simulink model "ArduinoDUE"  (R2024b)
settings: Solver=ode3  StartTime=0.0  StopTime=inf  RelTol=1e-3  EnableMultiTasking=on
libraries: arduinolib x7, simulink x5, arduinosensorlib x2, slpidlib x2
settings Model: SimulationMode=external  ExtModeTrigDuration=2  Creator=antho  LastModifiedBy=antho
settings SolverCC: AlgebraicLoopSolver=TrustRegion  AutoInsertRateTranBlk=on
settings DataIOCC: LimitDataPoints=on  SaveFormat=Array
settings OptimizationCC: ReuseModelBlockBuffer=off  ExpressionDepthLimit=2147483647  LifeSpan=Inf  MaxStackSize=64
settings DebuggingCC: UnderspecifiedInitializationDetection=Classic  MergeDetectMultiDrivingBlocksExec=none  FcnCallInpInsideContextMsg=warning  UnconnectedInputMsg=warning  UnconnectedOutputMsg=warning  UnconnectedLineMsg=warning  AllowSymbolicDim=off  StateNameClashWarn=warning  SFUnexpectedBacktrackingDiag=warning  SFNoUnconditionalDefaultTransitionDiag=warning  SFExecutionAtInitializationDiag=none  ArithmeticOperatorsInVariantConditions=warning
settings HardwareCC: ProdBitPerPointer=32  ProdBitPerSizeT=32  ProdBitPerPtrDiffT=32  ProdLargestAtomicInteger=Long  ProdLargestAtomicFloat=Double  ProdWordSize=32  ProdHWDeviceType=ARM Compatible->ARM Cortex
settings ModelReferenceCC: EnableRefExpFcnMdlSchedulingChecks=on  PropagateSignalLabelsOutOfModel=off
settings SFSimCC: SimUseLocalCustomCode=off  CustomCodeUndefinedFunction=UseInterfaceOnly
settings RTWCC: Description=Embedded Coder  SystemTargetFile=ert.tlc  HardwareBoard=Arduino Due  TemplateMakefile=ert_default_tmf  GenerateReport=on  RTWVerbose=off  RTWUseLocalCustomCode=off  Toolchain=Arduino ARM  BuildConfiguration=Faster Runs  LaunchReport=on  GPUComputeCapability=3.5
settings CodeAppCC: ForceParamTrailComments=on  OperatorAnnotations=on  StateflowObjectComments=on  MATLABSourceComments=on
settings ERTTargetCC: MultiwordLength=2048  ERTCustomFileBanners=off  SupportContinuousTime=on  SupportNonInlinedSFcns=on  RemoveResetFunc=off  SupportVariableSizeSignals=on  ModelStepFunctionPrototypeControlCompliant=off  ExtModeTransport=3  ExtModeStaticAlloc=on  ExtModeAutomaticAllocSize=off  ExtModeStaticAllocSize=24576  ExtModeMexFile=ext_xcp  ExtModeIntrfLevel=Level2 - Open  InlinedParameterPlacement=Hierarchical  DynamicArrayContainerType=coder::array
settings ConfigComp: CovMetricSettings=dw  CovSaveCumulativeToWorkspaceVar=on  CovSaveSingleToWorkspaceVar=on  CovExternalEMLEnable=off  CovSFcnEnable=off

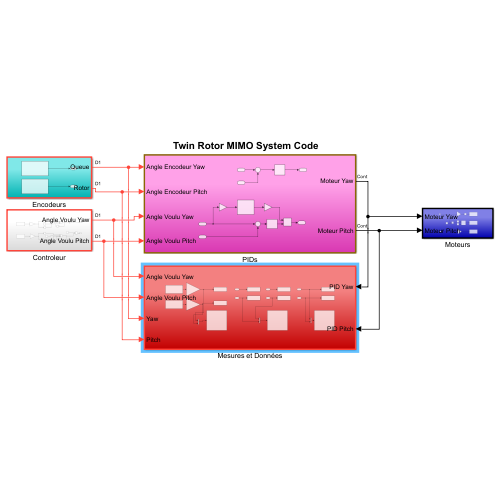
[thumbnail: Simulink's stored preview of the top-level diagram]
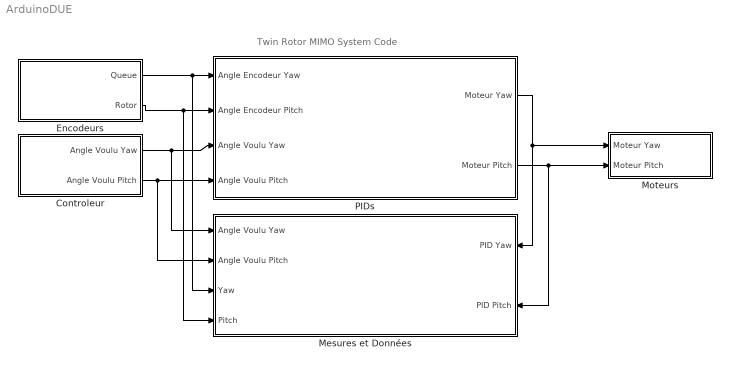
== system ArduinoDUE ==
  note: Twin Rotor MIMO System Code
  Controleur : Subsystem
  Encodeurs : Subsystem
  Mesures et Données : Subsystem
      settings: PortSchema="{\"entries\":[{\"content\":{\"sides\":[{\"content\":{\"connectorIds\":[\"In1\",\"In2\",\"In3\",\"In4\"]},\"type\":\"ConnectorPlacement.EquallySpacedRectSide\",\"uuid\":\"82e4522a-b4cd-44f9-a5c9-60d23544d279\"},{\"content\":{\"connectorIds\":[\"In5\",\"In6\"],\"side\":\"RIGHT\"},\"type\":\"ConnectorPlacement.EquallySpacedRectSide\",\"uuid\":\"29cf5c3e-0c08-4941-86a4-f83772340204\"},{\"content\":{\"side\":\"TOP\"},\"type\":\"ConnectorPlacement.EquallySpacedRectSide\",\"uuid\":\"e18b2821-c2fe-4315-852d-b03618fbc173\"}]},\"type\":\"ConnectorPlacement.EquallySpacedConnector\",\"uuid\":\"8888ef34-2317-47d3-9079-024b33e04ca1\"}],\"packageUris\":[\"http://schema.mathworks.com/mf0/Connector/R2020b\"],\"version\":\"1.0\"}"
  Moteurs : Subsystem
  PIDs : Subsystem
  wires:
  Encodeurs/1(Queue) -> Mesures et Données/3(Yaw), PIDs/1(Angle Encodeur Yaw)
  Encodeurs/2(Rotor) -> Mesures et Données/4(Pitch), PIDs/2(Angle Encodeur Pitch)
  Controleur/1(Angle Voulu Yaw) -> Mesures et Données/1(Angle Voulu Yaw), PIDs/3(Angle Voulu Yaw)
  Controleur/2(Angle Voulu Pitch) -> Mesures et Données/2(Angle Voulu Pitch), PIDs/4(Angle Voulu Pitch)
  PIDs/1(Moteur Yaw) -> Moteurs/1(Moteur Yaw), Mesures et Données/5(PID Yaw)
  PIDs/2(Moteur Pitch) -> Mesures et Données/6(PID Pitch), Moteurs/2(Moteur Pitch)

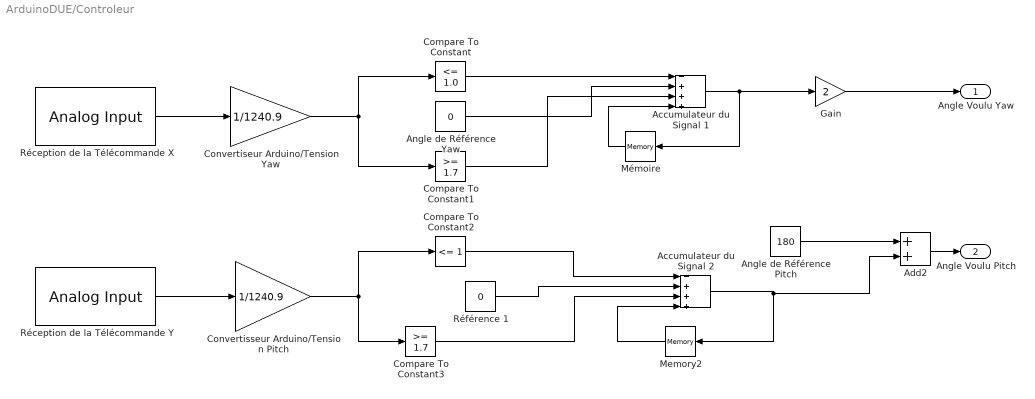
== system ArduinoDUE/Controleur ==
  Accumulateur du Signal 1 : Sum  Inputs=-+++
  Accumulateur du Signal 2 : Sum  Inputs=-+++
  Add2 : Sum
  Angle de Référence Pitch : Constant  Value=180
  Angle de Référence Yaw : Constant  Value=0
  Compare To Constant : simulink/Logic and Bit Operations/Compare To Constant  relop=<=  const=1.0  OutDataTypeStr=boolean
  Compare To Constant1 : simulink/Logic and Bit Operations/Compare To Constant  relop=>=  const=1.7  OutDataTypeStr=boolean
  Compare To Constant2 : simulink/Logic and Bit Operations/Compare To Constant  relop=<=  const=1  OutDataTypeStr=boolean
  Compare To Constant3 : simulink/Logic and Bit Operations/Compare To Constant  relop=>=  const=1.7  OutDataTypeStr=boolean
  Convertiseur Arduino/Tension Yaw : Gain  Gain=1/1240.9
  Convertisseur Arduino/Tension Pitch : Gain  Gain=1/1240.9
  Gain : Gain  Gain=2
  Memory2 : Memory
  Mémoire : Memory
  Réception de la Télécommande X : arduinolib/Analog Input  pinNumber=3  ReadResultsOnly=off  ConversionTriggerSource=Software  ExternalTriggerType=uint32( 0 )  OutputDataType=uint16  EnableConversionCompleteNotify=off  EnableOuputStatus=off  SampleTime=0.005  blockPlatform=arduino
  Réception de la Télécommande Y : arduinolib/Analog Input  pinNumber=4  ReadResultsOnly=off  ConversionTriggerSource=Software  ExternalTriggerType=uint32( 0 )  OutputDataType=uint16  EnableConversionCompleteNotify=off  EnableOuputStatus=off  SampleTime=0.005  blockPlatform=arduino
  Référence 1 : Constant  Value=0
  Angle Voulu Yaw : Outport
  Angle Voulu Pitch : Outport  Port=2
  wires:
  Convertiseur Arduino/Tension Yaw/1 -> Compare To Constant/1, Compare To Constant1/1
  Réception de la Télécommande Y/1 -> Convertisseur Arduino/Tension Pitch/1
  Convertisseur Arduino/Tension Pitch/1 -> Compare To Constant2/1, Compare To Constant3/1
  Réception de la Télécommande X/1 -> Convertiseur Arduino/Tension Yaw/1
  Accumulateur du Signal 1/1 -> Gain/1, Mémoire/1
  Angle de Référence Pitch/1 -> Add2/1
  Mémoire/1 -> Accumulateur du Signal 1/4
  Angle de Référence Yaw/1 -> Accumulateur du Signal 1/2
  Référence 1/1 -> Accumulateur du Signal 2/2
  Memory2/1 -> Accumulateur du Signal 2/4
  Accumulateur du Signal 2/1 -> Add2/2, Memory2/1
  Add2/1 -> Angle Voulu Pitch/1
  Compare To Constant/1 -> Accumulateur du Signal 1/1
  Compare To Constant2/1 -> Accumulateur du Signal 2/1
  Compare To Constant3/1 -> Accumulateur du Signal 2/3
  Compare To Constant1/1 -> Accumulateur du Signal 1/3
  Gain/1 -> Angle Voulu Yaw/1

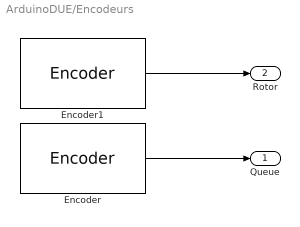
== system ArduinoDUE/Encodeurs ==
  Encoder : arduinosensorlib/Encoder  InputA=3  InputB=2  Mode=No reset  SampleTime=0.005
  Encoder1 : arduinosensorlib/Encoder  InputA=4  InputB=5  Mode=No reset  SampleTime=0.005
  Queue : Outport
  Rotor : Outport  Port=2
  wires:
  Encoder/1 -> Queue/1
  Encoder1/1 -> Rotor/1

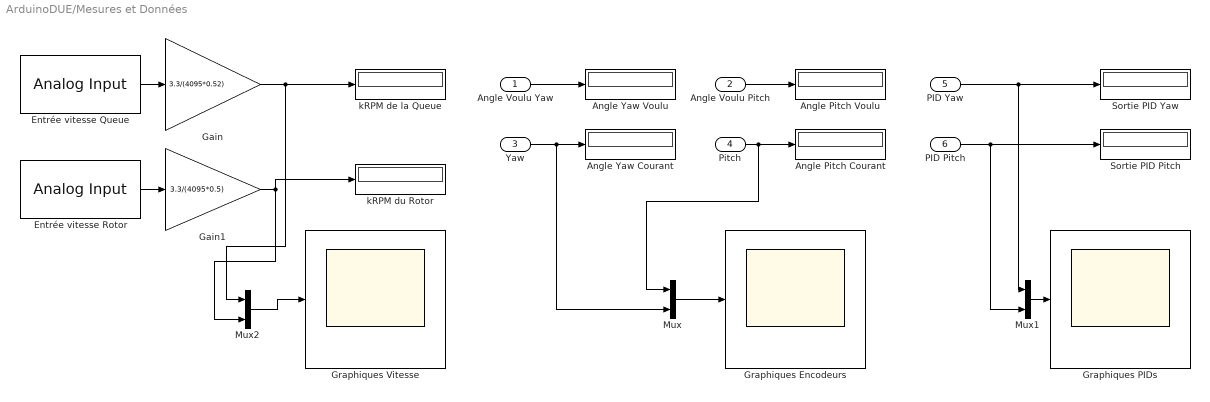
== system ArduinoDUE/Mesures et Données ==
  Angle Voulu Yaw : Inport
  Angle Voulu Pitch : Inport  Port=2
  Yaw : Inport  Port=3
  Pitch : Inport  Port=4
  PID Yaw : Inport  Port=5
  PID Pitch : Inport  Port=6
  Angle Pitch Courant : Display
  Angle Pitch Voulu : Display
  Angle Yaw Courant : Display
  Angle Yaw Voulu : Display
  Entrée vitesse Queue : arduinolib/Analog Input  pinNumber=2  ReadResultsOnly=off  ConversionTriggerSource=Software  ExternalTriggerType=uint32( 0 )  OutputDataType=uint16  EnableConversionCompleteNotify=off  EnableOuputStatus=off  SampleTime=0.005  blockPlatform=arduino
  Entrée vitesse Rotor : arduinolib/Analog Input  pinNumber=1  ReadResultsOnly=off  ConversionTriggerSource=Software  ExternalTriggerType=uint32( 0 )  OutputDataType=uint16  EnableConversionCompleteNotify=off  EnableOuputStatus=off  SampleTime=0.005  blockPlatform=arduino
  Gain : Gain  Gain=3.3/(4095*0.52)
  Gain1 : Gain  Gain=3.3/(4095*0.5)
  Graphiques Encodeurs : Scope
  Graphiques PIDs : Scope
  Graphiques Vitesse : Scope
  Mux : Mux  Inputs=2
  Mux1 : Mux  Inputs=2
  Mux2 : Mux  Inputs=2
  Sortie PID Pitch : Display
  Sortie PID Yaw : Display
  kRPM de la Queue : Display
  kRPM du Rotor : Display
  wires:
  Angle Voulu Yaw/1 -> Angle Yaw Voulu/1
  Yaw/1 -> Mux/2, Angle Yaw Courant/1
  Angle Voulu Pitch/1 -> Angle Pitch Voulu/1
  Pitch/1 -> Mux/1, Angle Pitch Courant/1
  PID Yaw/1 -> Mux1/1, Sortie PID Yaw/1
  PID Pitch/1 -> Mux1/2, Sortie PID Pitch/1
  Mux/1 -> Graphiques Encodeurs/1
  Entrée vitesse Queue/1 -> Gain/1
  Entrée vitesse Rotor/1 -> Gain1/1
  Mux1/1 -> Graphiques PIDs/1
  Mux2/1 -> Graphiques Vitesse/1
  Gain/1 -> Mux2/1, kRPM de la Queue/1
  Gain1/1 -> Mux2/2, kRPM du Rotor/1

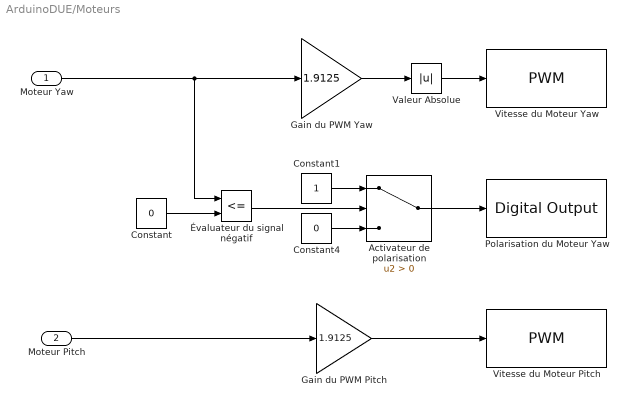
== system ArduinoDUE/Moteurs ==
  Moteur Yaw : Inport
  Moteur Pitch : Inport  Port=2
  Activateur de polarisation : Switch  Criteria=u2 > Threshold  SaturateOnIntegerOverflow=off  InputSameDT=off
  Constant : Constant  Value=0
  Constant1 : Constant
  Constant4 : Constant  Value=0
  Gain du PWM Pitch : Gain  Gain=1.9125
  Gain du PWM Yaw : Gain  Gain=1.9125
  Polarisation du Moteur Yaw : arduinolib/Digital Output  pinNumber=8  Direction=output  blockPlatform=arduino
  Valeur Absolue : Abs  SaturateOnIntegerOverflow=off
  Vitesse du Moteur Pitch : arduinolib/PWM  pinNumber=7  frequencyType=Specify  desiredFrequency=60  achievableFrequency=60
  Vitesse du Moteur Yaw : arduinolib/PWM  pinNumber=6  frequencyType=Specify  desiredFrequency=60  achievableFrequency=60
  Évaluateur du signal négatif : RelationalOperator  Operator=<=  OutDataTypeStr=boolean  RndMeth=Simplest  InputSameDT=off
  wires:
  Évaluateur du signal négatif/1 -> Activateur de polarisation/2
  Constant4/1 -> Activateur de polarisation/3
  Constant1/1 -> Activateur de polarisation/1
  Activateur de polarisation/1 -> Polarisation du Moteur Yaw/1
  Constant/1 -> Évaluateur du signal négatif/2
  Gain du PWM Yaw/1 -> Valeur Absolue/1
  Valeur Absolue/1 -> Vitesse du Moteur Yaw/1
  Moteur Yaw/1 -> Évaluateur du signal négatif/1, Gain du PWM Yaw/1
  Moteur Pitch/1 -> Gain du PWM Pitch/1
  Gain du PWM Pitch/1 -> Vitesse du Moteur Pitch/1

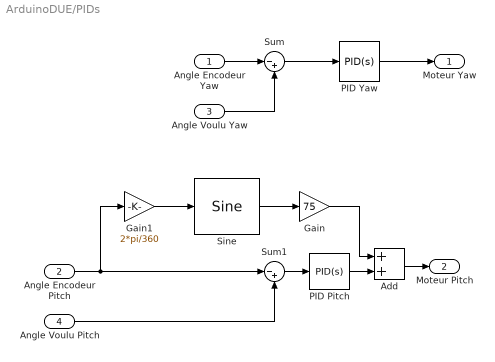
== system ArduinoDUE/PIDs ==
  Angle Encodeur Yaw : Inport
  Angle Encodeur Pitch : Inport  Port=2
  Angle Voulu Yaw : Inport  Port=3
  Angle Voulu Pitch : Inport  Port=4
  Add : Sum
  Gain : Gain  Gain=75
  Gain1 : Gain  Gain=2*pi/360
  PID Pitch : slpidlib/PID Controller  Controller=PID  Form=Parallel  TimeDomain=Continuous-time  UseExternalTs=off  SampleTime=-1  IntegratorMethod=Forward Euler  FilterMethod=Forward Euler  ControllerParametersSource=internal  P=4  I=0.4  UseKiTs=off  D=20  UseExternalDerivativeSource=off  N=100  UseFilter=on  TunerSelectOption=Transfer Function Based (PID Tuner App)  InitialConditionSource=internal  InitialConditionForIntegrator=0  InitialConditionForFilter=10000  DifferentiatorICPrevScaledInput=0  ExternalReset=none  TrackingMode=off  Kt=1  LimitOutput=off  SatLimitsSource=internal  UpperSaturationLimit=inf  LowerSaturationLimit=-inf  LinearizeAsGain=on  AntiWindupMode=none  Kb=1  LimitIntegrator=off  UpperIntegratorSaturationLimit=inf  LowerIntegratorSaturationLimit=-inf  POutMin=[]  POutMax=[]  IOutMin=[]  IOutMax=[]  DOutMin=[]  DOutMax=[]  NOutMin=[]  NOutMax=[]  SumOutMin=[]  SumOutMax=[]  SaturationOutMin=[]  SaturationOutMax=[]  PParamMin=[]  PParamMax=[]  IParamMin=[]  IParamMax=[]  DParamMin=[]  DParamMax=[]  NParamMin=[]  NParamMax=[]  KbParamMin=[]  KbParamMax=[]  KtParamMin=[]  KtParamMax=[]  KbOutMin=[]  KbOutMax=[]  KtOutMin=[]  KtOutMax=[]  IntegratorOutMin=[]  IntegratorOutMax=[]  FilterOutMin=[]  FilterOutMax=[]  SumI1OutMin=[]  SumI1OutMax=[]  SumI2OutMin=[]  SumI2OutMax=[]  SumI3OutMin=[]  SumI3OutMax=[]  SumI4OutMin=[]  SumI4OutMax=[]  SumDOutMin=[]  SumDOutMax=[]  DifferentiatorOutMin=[]  DifferentiatorOutMax=[]  FilterDiffOutCoefMin=[]  FilterDiffOutCoefMax=[]  ReciprocalOutMin=[]  ReciprocalOutMax=[]  SumDenOutMin=[]  SumDenOutMax=[]  SumNumOutMin=[]  SumNumOutMax=[]  DivideOutMin=[]  DivideOutMax=[]  UdiffTsProdOutMin=[]  UdiffTsProdOutMax=[]  NTsProdOutMin=[]  NTsProdOutMax=[]  UintegralTsProdOutMin=[]  UintegralTsProdOutMax=[]  UngainTsProdOutMin=[]  UngainTsProdOutMax=[]  ClampingZeroOutDataTypeStr=Inherit: Inherit via back propagation  ClampingZeroOutMin=[]  ClampingZeroOutMax=[]  FilterDenConstantOutDataTypeStr=Inherit: Inherit via back propagation  FilterDenConstantOutMin=[]  FilterDenConstantOutMax=[]  PCopyOutDataTypeStr=Inherit: Inherit via back propagation  PCopyOutMin=[]  PCopyOutMax=[]  NCopyOutDataTypeStr=Inherit: Inherit via back propagation  NCopyOutMin=[]  NCopyOutMax=[]  IntegratorContinuousStateAttributes=''  IntegratorStateMustResolveToSignalObject=off  IntegratorRTWStateStorageClass=Auto  FilterContinuousStateAttributes=''  FilterStateMustResolveToSignalObject=off  FilterRTWStateStorageClass=Auto  ParallelPVariant=InternalParameters  IdealPVariant=Disabled  IVariant=InternalParameters  DVariant=InternalParameters  IntegratorVariant=Continuous  SatVariant=Disabled  AWVariant=Passthrough  PCopyVariant=Disabled  TRVariant=Disabled  FdbkBlocksVariant=Forward  IdealPFdbkVariant=Disabled  SatFdbkVariant=Disabled  DerivativeFilterVariant=ContFilter  NVariant=InternalParameters  NCopyVariant=Disabled  FilterICVariant=InternalICsFilter  IntegratorICVariant=InternalICs  ExternalResetVariant=Disabled  TRSumVariant=Passthrough  SumFdbkVariant=Disabled  SumVariant=Sum_PID  TsampFilterVariant=InternalTs  TsampNgainVariant=Passthrough  TsampIntegralVariant=Disabled_SignalSpec  ExternalSaturationOutDataTypeStr=Inherit: Same as second input  DerivativeSourceVariant=ErrorSignal  PreIntVariant=InternalPreInt
  PID Yaw : slpidlib/PID Controller  Controller=PID  Form=Parallel  TimeDomain=Continuous-time  UseExternalTs=off  SampleTime=-1  IntegratorMethod=Forward Euler  FilterMethod=Forward Euler  ControllerParametersSource=internal  P=5  I=0.5  UseKiTs=off  D=20  UseExternalDerivativeSource=off  N=100  UseFilter=on  TunerSelectOption=Transfer Function Based (PID Tuner App)  InitialConditionSource=internal  InitialConditionForIntegrator=0  InitialConditionForFilter=10  DifferentiatorICPrevScaledInput=0  ExternalReset=none  TrackingMode=off  Kt=1  LimitOutput=off  SatLimitsSource=internal  UpperSaturationLimit=inf  LowerSaturationLimit=-inf  LinearizeAsGain=on  AntiWindupMode=none  Kb=1  LimitIntegrator=off  UpperIntegratorSaturationLimit=inf  LowerIntegratorSaturationLimit=-inf  POutMin=[]  POutMax=[]  IOutMin=[]  IOutMax=[]  DOutMin=[]  DOutMax=[]  NOutMin=[]  NOutMax=[]  SumOutMin=[]  SumOutMax=[]  SaturationOutMin=[]  SaturationOutMax=[]  PParamMin=[]  PParamMax=[]  IParamMin=[]  IParamMax=[]  DParamMin=[]  DParamMax=[]  NParamMin=[]  NParamMax=[]  KbParamMin=[]  KbParamMax=[]  KtParamMin=[]  KtParamMax=[]  KbOutMin=[]  KbOutMax=[]  KtOutMin=[]  KtOutMax=[]  IntegratorOutMin=[]  IntegratorOutMax=[]  FilterOutMin=[]  FilterOutMax=[]  SumI1OutMin=[]  SumI1OutMax=[]  SumI2OutMin=[]  SumI2OutMax=[]  SumI3OutMin=[]  SumI3OutMax=[]  SumI4OutMin=[]  SumI4OutMax=[]  SumDOutMin=[]  SumDOutMax=[]  DifferentiatorOutMin=[]  DifferentiatorOutMax=[]  FilterDiffOutCoefMin=[]  FilterDiffOutCoefMax=[]  ReciprocalOutMin=[]  ReciprocalOutMax=[]  SumDenOutMin=[]  SumDenOutMax=[]  SumNumOutMin=[]  SumNumOutMax=[]  DivideOutMin=[]  DivideOutMax=[]  UdiffTsProdOutMin=[]  UdiffTsProdOutMax=[]  NTsProdOutMin=[]  NTsProdOutMax=[]  UintegralTsProdOutMin=[]  UintegralTsProdOutMax=[]  UngainTsProdOutMin=[]  UngainTsProdOutMax=[]  ClampingZeroOutDataTypeStr=Inherit: Inherit via back propagation  ClampingZeroOutMin=[]  ClampingZeroOutMax=[]  FilterDenConstantOutDataTypeStr=Inherit: Inherit via back propagation  FilterDenConstantOutMin=[]  FilterDenConstantOutMax=[]  PCopyOutDataTypeStr=Inherit: Inherit via back propagation  PCopyOutMin=[]  PCopyOutMax=[]  NCopyOutDataTypeStr=Inherit: Inherit via back propagation  NCopyOutMin=[]  NCopyOutMax=[]  IntegratorContinuousStateAttributes=''  IntegratorStateMustResolveToSignalObject=off  IntegratorRTWStateStorageClass=Auto  FilterContinuousStateAttributes=''  FilterStateMustResolveToSignalObject=off  FilterRTWStateStorageClass=Auto  ParallelPVariant=InternalParameters  IdealPVariant=Disabled  IVariant=InternalParameters  DVariant=InternalParameters  IntegratorVariant=Continuous  SatVariant=Disabled  AWVariant=Passthrough  PCopyVariant=Disabled  TRVariant=Disabled  FdbkBlocksVariant=Forward  IdealPFdbkVariant=Disabled  SatFdbkVariant=Disabled  DerivativeFilterVariant=ContFilter  NVariant=InternalParameters  NCopyVariant=Disabled  FilterICVariant=InternalICsFilter  IntegratorICVariant=InternalICs  ExternalResetVariant=Disabled  TRSumVariant=Passthrough  SumFdbkVariant=Disabled  SumVariant=Sum_PID  TsampFilterVariant=InternalTs  TsampNgainVariant=Passthrough  TsampIntegralVariant=Disabled_SignalSpec  ExternalSaturationOutDataTypeStr=Inherit: Same as second input  DerivativeSourceVariant=ErrorSignal  PreIntVariant=InternalPreInt
  Sine : simulink/Lookup Tables/Sine  Formula=cos(2*pi*u)  NumDataPoints=(2^5)+1  OutputWordLength=16  InternalRulePriority=Speed
  Sum : Sum  Inputs=|-+
  Sum1 : Sum  Inputs=|-+
  Moteur Yaw : Outport
  Moteur Pitch : Outport  Port=2
  wires:
  Sum1/1 -> PID Pitch/1
  Angle Encodeur Yaw/1 -> Sum/1
  Angle Encodeur Pitch/1 -> Sum1/1, Gain1/1
  Angle Voulu Pitch/1 -> Sum1/2
  Angle Voulu Yaw/1 -> Sum/2
  PID Pitch/1 -> Add/2
  Gain1/1 -> Sine/1
  Sine/1 -> Gain/1
  Gain/1 -> Add/1
  Sum/1 -> PID Yaw/1
  PID Yaw/1 -> Moteur Yaw/1
  Add/1 -> Moteur Pitch/1
